simulink model "simulator"  (R2024a)
settings: Solver=FixedStepAuto  StartTime=0.0  StopTime=10  FixedStep=0.01  RelTol=1e-3
values from neighbouring files (symbols this model uses):
  beta2 = 5    [Evaluation.m]    (also in step_by_step.m = 1)
  beta3 = 5    [Evaluation.m]    (also in step_by_step.m = 1)
  g = 10    [Evaluation.m]    (also in step_by_step.m)
  initial_x1 = sorted_x(2)    [Evaluation.m]    (also in step_by_step.m)
  initial_x2 = sorted_x(3)    [Evaluation.m]    (also in step_by_step.m)
  initial_y1 = sorted_y(2)    [Evaluation.m]    (also in step_by_step.m)
  initial_y2 = sorted_y(3)    [Evaluation.m]    (also in step_by_step.m)
  k2 = 40    [step_by_step.m]
  k3 = 10    [step_by_step.m]
  Lr1 = sqrt((initial_x1 - ref_x)^2 + (initial_y1 - ref_y)^2)    [Evaluation.m]    (also in step_by_step.m)
  Lr2 = sqrt((initial_x2 - ref_x)^2 + (initial_y2 - ref_y)^2)    [Evaluation.m]    (also in step_by_step.m)
  Lr3 = sqrt((initial_x1 - initial_x2)^2 + (initial_y1 - initial_y2)^2)    [Evaluation.m]    (also in step_by_step.m)
  m1 = 1    [Evaluation.m]    (also in step_by_step.m)
  m2 = 1    [Evaluation.m]    (also in step_by_step.m)
  ref_x = sorted_x(1)    [Evaluation.m]    (also in step_by_step.m)
  ref_y = sorted_y(1)    [Evaluation.m]    (also in step_by_step.m)
undefined symbols (not defined in the file or in its folder): beta1, k1
settings Model: Creator=lucid  LastModifiedBy=lucid

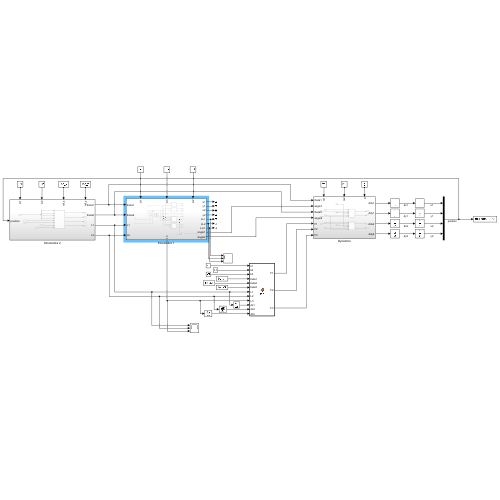
[thumbnail: Simulink's stored preview of the top-level diagram]
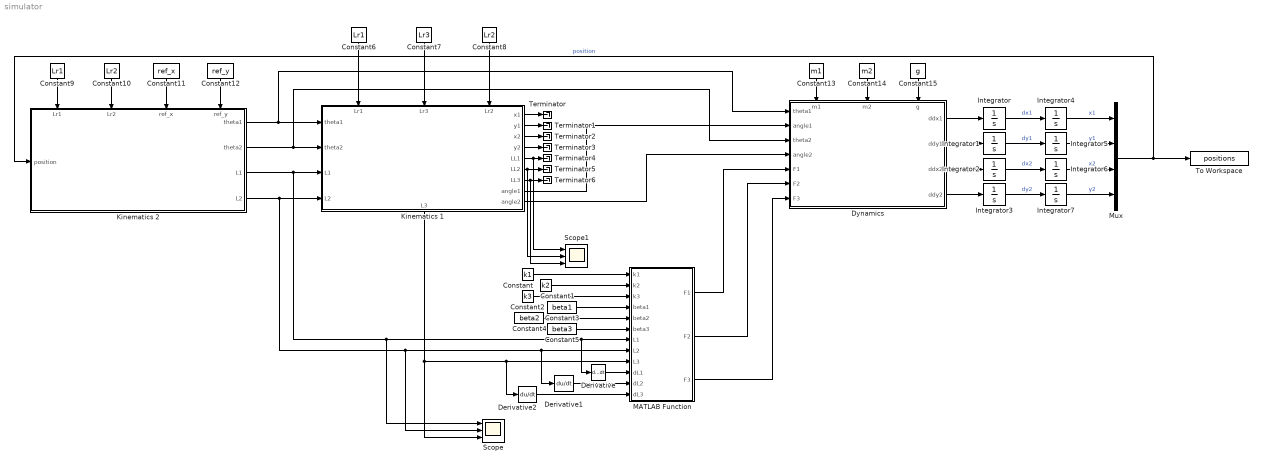
== system simulator ==
  Constant : Constant  Value=k1
  Constant1 : Constant  Value=k2
  Constant10 : Constant  Value=Lr2
  Constant11 : Constant  Value=ref_x
  Constant12 : Constant  Value=ref_y
  Constant13 : Constant  Value=m1
  Constant14 : Constant  Value=m2
  Constant15 : Constant  Value=g
  Constant2 : Constant  Value=k3
  Constant3 : Constant  Value=beta1
  Constant4 : Constant  Value=beta2
  Constant5 : Constant  Value=beta3
  Constant6 : Constant  Value=Lr1
  Constant7 : Constant  Value=Lr3
  Constant8 : Constant  Value=Lr2
  Constant9 : Constant  Value=Lr1
  Derivative : Derivative
  Derivative1 : Derivative
  Derivative2 : Derivative
  Dynamics : Subsystem
      settings: PortSchema="{\"entries\":[{\"content\":{\"sides\":[{\"content\":{\"connectorIds\":[\"In1\",\"In2\",\"In3\",\"In4\",\"In5\",\"In6\",\"In7\"]},\"type\":\"ConnectorPlacement.EquallySpacedRectSide\",\"uuid\":\"5b94e20a-9cf5-4f9d-9248-6bb3e57fc93a\"},{\"content\":{\"connectorIds\":[\"Out1\",\"Out2\",\"Out3\",\"Out4\"],\"side\":\"RIGHT\"},\"type\":\"ConnectorPlacement.EquallySpacedRectSide\",\"uuid\":\"4e8619a1-46fd-442d-b05b-54a4d8ffe983\"},{\"content\":{\"connectorIds\":[\"In8\",\"In9\",\"In10\"],\"side\":\"TOP\"},\"type\":\"ConnectorPlacement.EquallySpacedRectSide\",\"uuid\":\"35018220-2ddc-42be-8e11-f84a93551bf0\"}]},\"type\":\"ConnectorPlacement.EquallySpacedConnector\",\"uuid\":\"aac71a47-7196-4a0b-9832-3bbc03ebde8e\"}],\"packageUris\":[\"http://schema.mathworks.com/mf0/Connector/R2020b\"],\"version\":\"1.0\"}"
  Integrator{,1..3} (4 alike) : Integrator
  Integrator4 : Integrator  InitialCondition=initial_x1
  Integrator5 : Integrator  InitialCondition=initial_y1
  Integrator6 : Integrator  InitialCondition=initial_x2
  Integrator7 : Integrator  InitialCondition=initial_y2
  Kinematics 1 : Subsystem
      settings: PortSchema="{\"entries\":[{\"content\":{\"sides\":[{\"content\":{\"connectorIds\":[\"In1\",\"In2\",\"In3\",\"In4\"]},\"type\":\"ConnectorPlacement.EquallySpacedRectSide\",\"uuid\":\"3c5545fa-d53a-4f16-a033-6cd12df3b5c9\"},{\"content\":{\"connectorIds\":[\"Out1\",\"Out2\",\"Out3\",\"Out4\",\"Out5\",\"Out6\",\"Out7\",\"Out8\",\"Out9\"],\"side\":\"RIGHT\"},\"type\":\"ConnectorPlacement.EquallySpacedRectSide\",\"uuid\":\"0d9534c5-ddd5-4978-9644-9b9fc6951eaa\"},{\"content\":{\"connectorIds\":[\"In5\",\"In6\",\"In7\"],\"side\":\"TOP\"},\"type\":\"ConnectorPlacement.EquallySpacedRectSide\",\"uuid\":\"76b6e756-8e29-43c0-bffb-5b24a01ef5bc\"},{\"content\":{\"connectorIds\":[\"Out10\"],\"side\":\"BOTTOM\"},\"type\":\"ConnectorPlacement.EquallySpacedRectSide\",\"uuid\":\"e2f70fdc-c5a6-4688-9f0a-f203b03402a1\"}]},\"type\":\"ConnectorPlacement.EquallySpacedConnector\",\"uuid\":\"3b9442dd-21c4-47cf-ab63-ff7a081f600e\"}],\"packageUris\":[\"http://schema.mathworks.com/mf0/Connector/R2020b\"],\"version\":\"1.0\"}"
  Kinematics 2 : Subsystem
      settings: PortSchema="{\"entries\":[{\"content\":{\"sides\":[{\"content\":{\"connectorIds\":[\"In1\"]},\"type\":\"ConnectorPlacement.EquallySpacedRectSide\",\"uuid\":\"f7d693f2-e773-4e9f-aff4-690a43ff875b\"},{\"content\":{\"connectorIds\":[\"Out1\",\"Out2\",\"Out3\",\"Out4\"],\"side\":\"RIGHT\"},\"type\":\"ConnectorPlacement.EquallySpacedRectSide\",\"uuid\":\"467929e0-bb28-4c29-923e-093df099761e\"},{\"content\":{\"connectorIds\":[\"In2\",\"In3\",\"In4\",\"In5\"],\"side\":\"TOP\"},\"type\":\"ConnectorPlacement.EquallySpacedRectSide\",\"uuid\":\"7fcf5156-ea8a-4bcc-bff6-adea27895fb6\"}]},\"type\":\"ConnectorPlacement.EquallySpacedConnector\",\"uuid\":\"cb5239eb-5729-429b-aded-7e946fad81fd\"}],\"packageUris\":[\"http://schema.mathworks.com/mf0/Connector/R2020b\"],\"version\":\"1.0\"}"
  MATLAB Function : MATLAB Function  TreatAsAtomicUnit=on
  Mux : Mux
  Scope : Scope  NumInputPorts=3
  Scope1 : Scope  NumInputPorts=3
  Terminator{,1..6} (7 alike) : Terminator
  To Workspace : ToWorkspace  VariableName=positions  SaveFormat=Structure With Time  SampleTime=-1
  wires:
  Kinematics 2/2(theta2) -> Dynamics/3(theta2), Kinematics 1/2(theta2)
  Kinematics 2/4(L2) -> Scope/2, MATLAB Function/8(L2), Derivative1/1, Kinematics 1/4(L2)
  Kinematics 2/1(theta1) -> Dynamics/1(theta1), Kinematics 1/1(theta1)
  Kinematics 1/8(angle1) -> Dynamics/2(angle1)
  Kinematics 1/9(angle2) -> Dynamics/4(angle2)
  MATLAB Function/1(F1) -> Dynamics/5(F1)
  MATLAB Function/2(F2) -> Dynamics/6(F2)
  MATLAB Function/3(F3) -> Dynamics/7(F3)
  Kinematics 1/10(L3) -> Scope/3, Derivative2/1, MATLAB Function/9(L3)
  Derivative/1 -> MATLAB Function/10(dL1)
  Kinematics 2/3(L1) -> Scope/1, Derivative/1, MATLAB Function/7(L1), Kinematics 1/3(L1)
  Derivative1/1 -> MATLAB Function/11(dL2)
  Derivative2/1 -> MATLAB Function/12(dL3)
  Dynamics/1(ddx1) -> Integrator/1
  Dynamics/2(ddy1) -> Integrator1/1
  Dynamics/3(ddx2) -> Integrator2/1
  Dynamics/4(ddy2) -> Integrator3/1
  Integrator/1 -> Integrator4/1  "dx1"
  Integrator3/1 -> Integrator7/1  "dy2"
  Integrator2/1 -> Integrator6/1  "dx2"
  Integrator1/1 -> Integrator5/1  "dy1"
  Integrator4/1 -> Mux/1  "x1"
  Integrator5/1 -> Mux/2  "y1"
  Integrator6/1 -> Mux/3  "x2"
  Integrator7/1 -> Mux/4  "y2"
  Mux/1 -> To Workspace/1, Kinematics 2/1(position)  "position"
  Kinematics 1/1(x1) -> Terminator/1
  Kinematics 1/2(y1) -> Terminator1/1
  Kinematics 1/3(x2) -> Terminator2/1
  Kinematics 1/4(y2) -> Terminator3/1
  Kinematics 1/5(LL1) -> Scope1/1, Terminator4/1
  Kinematics 1/6(LL2) -> Scope1/2, Terminator5/1
  Kinematics 1/7("LL3 ") -> Scope1/3, Terminator6/1
  Constant/1 -> MATLAB Function/1(k1)
  Constant1/1 -> MATLAB Function/2(k2)
  Constant2/1 -> MATLAB Function/3(k3)
  Constant3/1 -> MATLAB Function/4(beta1)
  Constant4/1 -> MATLAB Function/5(beta2)
  Constant5/1 -> MATLAB Function/6(beta3)
  Constant13/1 -> Dynamics/8(m1)
  Constant14/1 -> Dynamics/9(m2)
  Constant15/1 -> Dynamics/10(g)
  Constant9/1 -> Kinematics 2/2(Lr1)
  Constant6/1 -> Kinematics 1/5(Lr1)
  Constant10/1 -> Kinematics 2/3(Lr2)
  Constant8/1 -> Kinematics 1/7(Lr2)
  Constant7/1 -> Kinematics 1/6(Lr3)
  Constant11/1 -> Kinematics 2/4(ref_x)
  Constant12/1 -> Kinematics 2/5(ref_y)

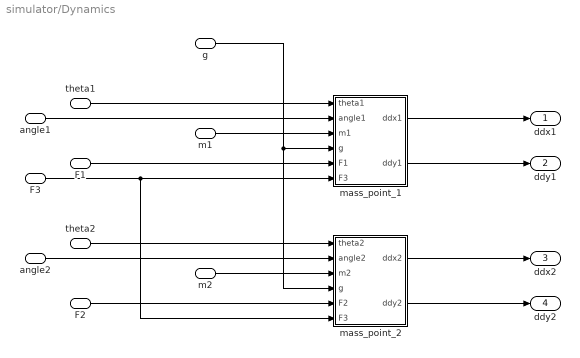
== system simulator/Dynamics ==
  theta1 : Inport
  angle1 : Inport  Port=2
  theta2 : Inport  Port=3
  angle2 : Inport  Port=4
  F1 : Inport  Port=5
  F2 : Inport  Port=6
  F3 : Inport  Port=7
  m1 : Inport  Port=8
  m2 : Inport  Port=9
  g : Inport  Port=10
  mass_point_1 : MATLAB Function  TreatAsAtomicUnit=on
  mass_point_2 : MATLAB Function  TreatAsAtomicUnit=on
  ddx1 : Outport
  ddy1 : Outport  Port=2
  ddx2 : Outport  Port=3
  ddy2 : Outport  Port=4
  wires:
  mass_point_1/1(ddx1) -> ddx1/1
  mass_point_1/2(ddy1) -> ddy1/1
  mass_point_2/1(ddx2) -> ddx2/1
  mass_point_2/2(ddy2) -> ddy2/1
  theta1/1 -> mass_point_1/1(theta1)
  angle1/1 -> mass_point_1/2(angle1)
  theta2/1 -> mass_point_2/1(theta2)
  angle2/1 -> mass_point_2/2(angle2)
  F1/1 -> mass_point_1/5(F1)
  F3/1 -> mass_point_1/6(F3), mass_point_2/6(F3)
  F2/1 -> mass_point_2/5(F2)
  m1/1 -> mass_point_1/3(m1)
  m2/1 -> mass_point_2/3(m2)
  g/1 -> mass_point_2/4(g), mass_point_1/4(g)

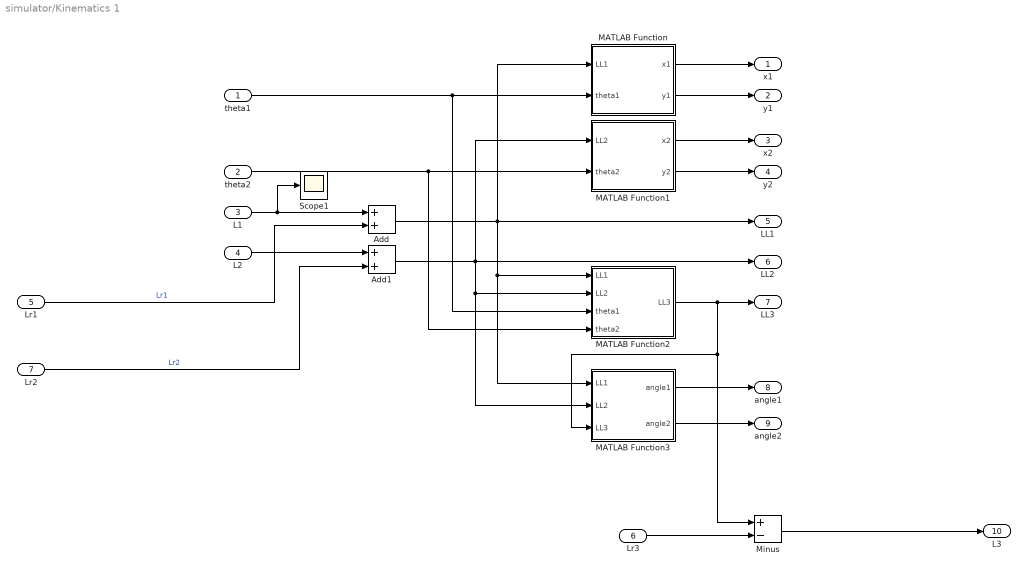
== system simulator/Kinematics 1 ==
  theta1 : Inport
  theta2 : Inport  Port=2
  L1 : Inport  Port=3
  L2 : Inport  Port=4
  Lr1 : Inport  Port=5
  Lr3 : Inport  Port=6
  Lr2 : Inport  Port=7
  Add : Sum
  Add1 : Sum
  MATLAB Function : MATLAB Function  TreatAsAtomicUnit=on
  MATLAB Function1 : MATLAB Function  TreatAsAtomicUnit=on
  MATLAB Function2 : MATLAB Function  TreatAsAtomicUnit=on
  MATLAB Function3 : MATLAB Function  TreatAsAtomicUnit=on
  Minus : Sum  Inputs=+-
  Scope1 : Scope
  x1 : Outport
  y1 : Outport  Port=2
  x2 : Outport  Port=3
  y2 : Outport  Port=4
  LL1 : Outport  Port=5
  LL2 : Outport  Port=6
  "LL3 " : Outport  Port=7
  angle1 : Outport  Port=8
  angle2 : Outport  Port=9
  L3 : Outport  Port=10
  wires:
  Lr1/1 -> Add/2  "Lr1"
  Lr2/1 -> Add1/2  "Lr2"
  Add/1 -> MATLAB Function3/1(LL1), MATLAB Function2/1(LL1), MATLAB Function/1(LL1), LL1/1
  L1/1 -> Scope1/1, Add/1
  Add1/1 -> MATLAB Function3/2(LL2), MATLAB Function2/2(LL2), MATLAB Function1/1(LL2), LL2/1
  L2/1 -> Add1/1
  MATLAB Function/1(x1) -> x1/1
  MATLAB Function/2(y1) -> y1/1
  theta1/1 -> MATLAB Function2/3(theta1), MATLAB Function/2(theta1)
  MATLAB Function1/2(y2) -> y2/1
  MATLAB Function1/1(x2) -> x2/1
  theta2/1 -> MATLAB Function2/4(theta2), MATLAB Function1/2(theta2)
  MATLAB Function2/1(LL3) -> Minus/1, MATLAB Function3/3(LL3), "LL3 "/1
  MATLAB Function3/1(angle1) -> angle1/1
  MATLAB Function3/2(angle2) -> angle2/1
  Minus/1 -> L3/1
  Lr3/1 -> Minus/2

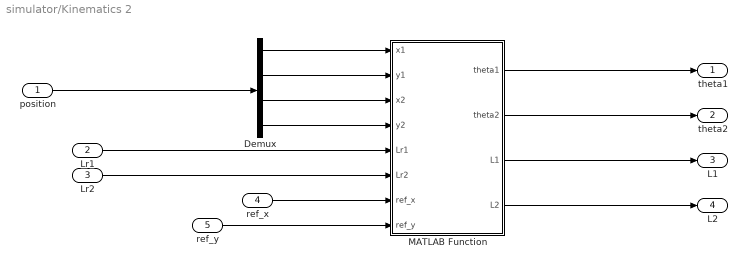
== system simulator/Kinematics 2 ==
  position : Inport
  Lr1 : Inport  Port=2
  Lr2 : Inport  Port=3
  ref_x : Inport  Port=4
  ref_y : Inport  Port=5
  Demux : Demux
  MATLAB Function : MATLAB Function  TreatAsAtomicUnit=on
  theta1 : Outport
  theta2 : Outport  Port=2
  L1 : Outport  Port=3
  L2 : Outport  Port=4
  wires:
  MATLAB Function/4(L2) -> L2/1
  MATLAB Function/3(L1) -> L1/1
  MATLAB Function/2(theta2) -> theta2/1
  MATLAB Function/1(theta1) -> theta1/1
  Demux/1 -> MATLAB Function/1(x1)
  Demux/2 -> MATLAB Function/2(y1)
  Demux/3 -> MATLAB Function/3(x2)
  Demux/4 -> MATLAB Function/4(y2)
  position/1 -> Demux/1
  Lr1/1 -> MATLAB Function/5(Lr1)
  Lr2/1 -> MATLAB Function/6(Lr2)
  ref_x/1 -> MATLAB Function/7(ref_x)
  ref_y/1 -> MATLAB Function/8(ref_y)

== matlab function simulator/Kinematics 2/MATLAB Function ==
  data: x1 input; theta1 output; theta2 output; L1 output; L2 output; y1 input; x2 input; y2 input; Lr1 input; Lr2 input; ref_x input; ref_y input
function [theta1,theta2,L1,L2] = fcn(x1,y1,x2,y2,Lr1,Lr2,ref_x,ref_y)

LL1 = sqrt((x1 - ref_x) ^2 + (y1 - ref_y) ^ 2);
L1 = LL1 - Lr1;

LL2 = sqrt((x2 - ref_x) ^2 + (y2 - ref_y) ^ 2);
L2 = LL2 - Lr2;

theta1 = atan2(x1-ref_x, -(y1-ref_y));
theta2 = atan2(x2-ref_x,- (y2-ref_y));

== matlab function simulator/Kinematics 1/MATLAB Function1 ==
  data: LL2 input; x2 output; theta2 input; y2 output
function [x2, y2]= fcn(LL2, theta2)


x2 = LL2 * sin(theta2);

y2 = - LL2 * cos(theta2);

== matlab function simulator/Kinematics 1/MATLAB Function ==
  data: LL1 input; x1 output; theta1 input; y1 output
function [x1, y1]= fcn(LL1, theta1)


x1 = LL1 * sin(theta1);

y1 = - LL1 * cos(theta1);

== matlab function simulator/Kinematics 1/MATLAB Function2 ==
  data: LL1 input; LL2 input; theta1 input; LL3 output; theta2 input
function LL3 = fcn(LL1, LL2, theta1, theta2)


theta = theta2 - theta1;

LL3 = sqrt(LL1^2 + LL2^2 - 2 * LL1 * LL2 * cos(theta));

== matlab function simulator/Kinematics 1/MATLAB Function3 ==
  data: LL1 input; LL2 input; LL3 input; angle1 output; angle2 output
function [angle1, angle2] = fcn(LL1,LL2,LL3)

cosAngle1 = (LL1^2 + LL3^2 - LL1^2) / (2 * LL1 * LL3);
cosAngle2 = (LL2^2 + LL3^2 - LL2^2) / (2 * LL2 * LL3);

angle1 = acos(cosAngle1);
angle2 = acos(cosAngle2);

== matlab function simulator/Dynamics/mass_point_1 ==
  data: theta1 input; ddx1 output; ddy1 output; angle1 input; m1 input; g input; F1 input; F3 input
function [ddx1,ddy1] = fcn(theta1,angle1,m1,g,F1,F3)

ddy1 = 1/m1 * (F1 * cos(theta1) + F3 * cos(-theta1 + angle1) - m1 * g);

ddx1 = 1/m1 * (F1 * (- sin(theta1)) + F3 * sin(-theta1 + angle1));

== matlab function simulator/Dynamics/mass_point_2 ==
  data: theta2 input; ddx2 output; ddy2 output; angle2 input; m2 input; g input; F2 input; F3 input
function [ddx2,ddy2] = fcn(theta2,angle2,m2,g,F2,F3)

ddy2 = 1/m2 * (F2 * cos(theta2) + F3 * cos(theta2 + angle2) - m2 * g);

ddx2 = 1/m2 * (- F2 * sin(theta2) - F3 * sin(theta2 + angle2));

== matlab function simulator/MATLAB Function ==
  data: k1 input; F1 output; F2 output; F3 output; k2 input; k3 input; beta1 input; beta2 input; beta3 input; L1 input; L2 input; L3 input; dL1 input; dL2 input; dL3 input
function [F1,F2,F3] = fcn(k1,k2,k3,beta1,beta2,beta3,L1,L2,L3,dL1,dL2,dL3)

F1 = k1 * L1 + beta1 * dL1;

F2 = k2 * L2 + beta2 * dL2;

F3 = k3 * L3 + beta3 * dL3;
